simulink model "Circuit2_tryingtoswitchthesystem"  (R2018b)
settings: Solver=ode4  StartTime=0.0  StopTime=5  FixedStep=1e-4  RelTol=1e-3
values from neighbouring files (symbols this model uses):
  Be = 1300e6    (= 1300000000)    [Circuit1_load.m]    (also in Circuit2_values.m)
  BeA = 1200e6    (= 1200000000)    [Circuit2_values.m]    (also in Circut3_values.m = 1300000000)
  BeB = 1500e6    (= 1500000000)    [Circuit2_values.m]    (also in Circut3_values.m = 1300000000)
  Cd = 0.7    [Circuit1_load.m]    (also in Circuit2_values.m)
  Dorifice = 2e-2    (= 0.02)    [Circuit1_load.m]    (also in Circuit2_values.m = 0.004)
  Dspool = 1e-2    (= 0.01)    [Circuit2_values.m]
  Kp = (1.e-3)/(10e5)    (= 1e-09)    [Circuit1_load.m]    (also in Circuit2_values.m; Circut3_values.m)
  pref = 180e5    (= 18000000)    [Circuit1_load.m]    (also in Circuit2_values.m; Circut3_values.m = 17000000)
  rho = 860    [Circuit1_load.m]    (also in Circuit2_values.m; Circut3_values.m)
  tau = 60e-3    (= 0.06)    [Circuit1_load.m]    (also in Circuit2_values.m = 0.03)
  V = 3e-3    (= 0.003)    [Circuit1_load.m]    (also in Circuit2_values.m)
  VA = 5e-4    (= 0.0005)    [Circuit2_values.m]    (also in Circut3_values.m = 0.0015)
  VB = 5e-4    (= 0.0005)    [Circuit2_values.m]    (also in Circut3_values.m = 0.003)
settings Model: Creator=Janne  LastModifiedBy=Janne

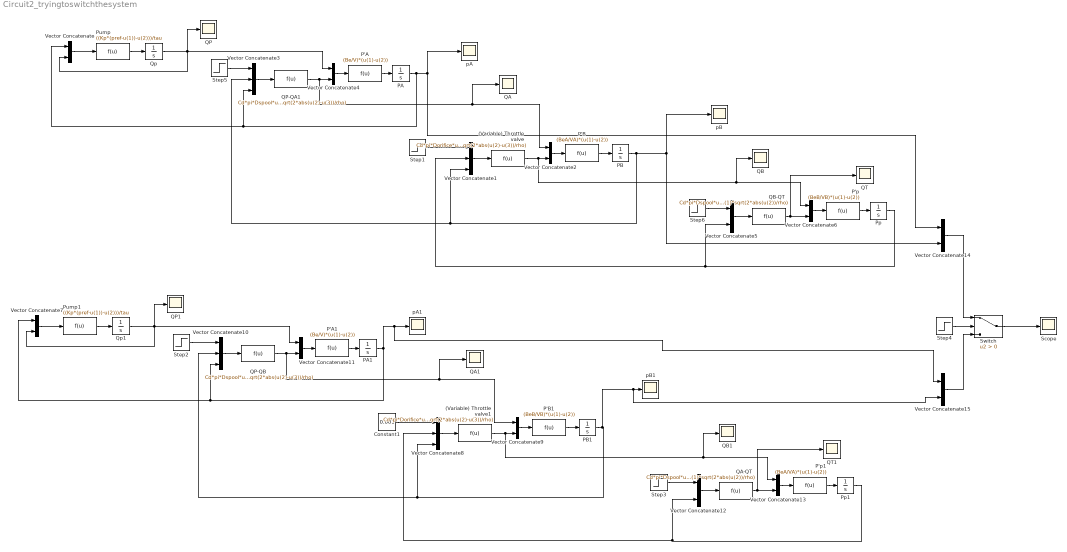
== system Circuit2_tryingtoswitchthesystem ==
  (Variable) Throttle valve : Fcn  Expr=Cd*pi*Dorifice*u(1)*sqrt(2*abs(u(2)-u(3))/rho)
  (Variable) Throttle valve1 : Fcn  Expr=Cd*pi*Dorifice*u(1)*sqrt(2*abs(u(2)-u(3))/rho)
  Constant1 : Constant  Value=0.001
  P'A : Fcn  Expr=(Be/V)*(u(1)-u(2))
  P'A1 : Fcn  Expr=(Be/V)*(u(1)-u(2))
  P'B : Fcn  Expr=(BeA/VA)*(u(1)-u(2))
  P'B1 : Fcn  Expr=(BeB/VB)*(u(1)-u(2))
  P'p : Fcn  Expr=(BeB/VB)*(u(1)-u(2))
  P'p1 : Fcn  Expr=(BeA/VA)*(u(1)-u(2))
  PA : Integrator  LimitOutput=on  UpperSaturationLimit=1000e5  LowerSaturationLimit=0
  PA1 : Integrator  LimitOutput=on  UpperSaturationLimit=1000e5  LowerSaturationLimit=0
  PB : Integrator  LimitOutput=on  UpperSaturationLimit=1000e5  LowerSaturationLimit=0
  PB1 : Integrator  LimitOutput=on  UpperSaturationLimit=1000e5  LowerSaturationLimit=0
  Pp : Integrator  LimitOutput=on  UpperSaturationLimit=1000e5  LowerSaturationLimit=0
  Pp1 : Integrator  LimitOutput=on  UpperSaturationLimit=1000e5  LowerSaturationLimit=0
  Pump : Fcn  Expr=((Kp*(pref-u(1))-u(2)))/tau
  Pump1 : Fcn  Expr=((Kp*(pref-u(1))-u(2)))/tau
  QA : Scope
  QA-QT : Fcn  Expr=Cd*pi*Dspool*u(1)*sqrt(2*abs(u(2))/rho)
  QA1 : Scope
  QB : Scope
  QB-QT : Fcn  Expr=Cd*pi*Dspool*u(1)*sqrt(2*abs(u(2))/rho)
  QB1 : Scope
  QP : Scope
  QP-QA1 : Fcn  Expr=Cd*pi*Dspool*u(1)*sqrt(2*abs(u(2)-u(3))/rho)
  QP-QB : Fcn  Expr=Cd*pi*Dspool*u(1)*sqrt(2*abs(u(2)-u(3))/rho)
  QP1 : Scope
  QT : Scope
  QT1 : Scope
  Qp : Integrator  LimitOutput=on  UpperSaturationLimit=1000e5  LowerSaturationLimit=0
  Qp1 : Integrator  LimitOutput=on  UpperSaturationLimit=1000e5  LowerSaturationLimit=0
  Scope : Scope
  Step1 : Step  Time=2  Before=0.0004  After=0  SampleTime=0
  Step2 : Step  Time=2  After=0.0004  SampleTime=0
  Step3 : Step  Time=2  After=0.0004  SampleTime=0
  Step4 : Step  Time=2  Before=0.0004  After=0.0004  SampleTime=0
  Step5 : Step  Time=2  Before=0.0004  After=0  SampleTime=0
  Step6 : Step  Time=2  Before=0.0004  After=0  SampleTime=0
  Switch : Switch  Criteria=u2 > Threshold
  Vector Concatenate{,2,4..7,9,11..15} (12 alike) : Concatenate
  Vector Concatenate{1,3,8,10} (4 alike) : Concatenate  NumInputs=3
  pA : Scope
  pA1 : Scope
  pB : Scope
  pB1 : Scope
  wires:
  Pump/1 -> Qp/1
  Vector Concatenate/1 -> Pump/1
  Vector Concatenate1/1 -> (Variable) Throttle valve/1
  Step1/1 -> Vector Concatenate1/1
  Vector Concatenate2/1 -> P'B/1
  P'B/1 -> PB/1
  Qp/1 -> Vector Concatenate/2, QP/1, Vector Concatenate4/1
  QP-QA1/1 -> QA/1, Vector Concatenate2/1, Vector Concatenate4/2
  Vector Concatenate4/1 -> P'A/1
  Vector Concatenate3/1 -> QP-QA1/1
  P'A/1 -> PA/1
  Step5/1 -> Vector Concatenate3/1
  PA/1 -> Vector Concatenate/1, Vector Concatenate3/3, Vector Concatenate14/1, pA/1
  Step6/1 -> Vector Concatenate5/1
  P'p/1 -> Pp/1
  Vector Concatenate5/1 -> QB-QT/1
  Vector Concatenate6/1 -> P'p/1
  QB-QT/1 -> Vector Concatenate6/2, QT/1
  (Variable) Throttle valve/1 -> QB/1, Vector Concatenate6/1, Vector Concatenate2/2
  Pp/1 -> Vector Concatenate1/2, Vector Concatenate5/2
  PB/1 -> pB/1, Vector Concatenate14/2, Vector Concatenate3/2, Vector Concatenate1/3
  Step4/1 -> Switch/2
  Vector Concatenate14/1 -> Switch/1
  QP-QB/1 -> QA1/1, Vector Concatenate9/1, Vector Concatenate11/2
  (Variable) Throttle valve1/1 -> QB1/1, Vector Concatenate13/1, Vector Concatenate9/2
  Vector Concatenate13/1 -> P'p1/1
  Step2/1 -> Vector Concatenate10/1
  PB1/1 -> Vector Concatenate15/2, pB1/1, Vector Concatenate10/2, Vector Concatenate8/3
  Pump1/1 -> Qp1/1
  QA-QT/1 -> Vector Concatenate13/2, QT1/1
  PA1/1 -> Vector Concatenate15/1, pA1/1, Vector Concatenate7/1, Vector Concatenate10/3
  Vector Concatenate11/1 -> P'A1/1
  Qp1/1 -> Vector Concatenate7/2, QP1/1, Vector Concatenate11/1
  Pp1/1 -> Vector Concatenate8/2, Vector Concatenate12/2
  P'B1/1 -> PB1/1
  P'A1/1 -> PA1/1
  P'p1/1 -> Pp1/1
  Vector Concatenate10/1 -> QP-QB/1
  Step3/1 -> Vector Concatenate12/1
  Vector Concatenate9/1 -> P'B1/1
  Vector Concatenate8/1 -> (Variable) Throttle valve1/1
  Vector Concatenate7/1 -> Pump1/1
  Constant1/1 -> Vector Concatenate8/1
  Vector Concatenate12/1 -> QA-QT/1
  Vector Concatenate15/1 -> Switch/3
  Switch/1 -> Scope/1
